simulink model "lesson140313_22"  (R2013a)
settings: Solver=ode45  StartTime=0.0  StopTime=10.0  RelTol=1e-3
settings Model: Creator=mulleda2  LastModifiedBy=mulleda2

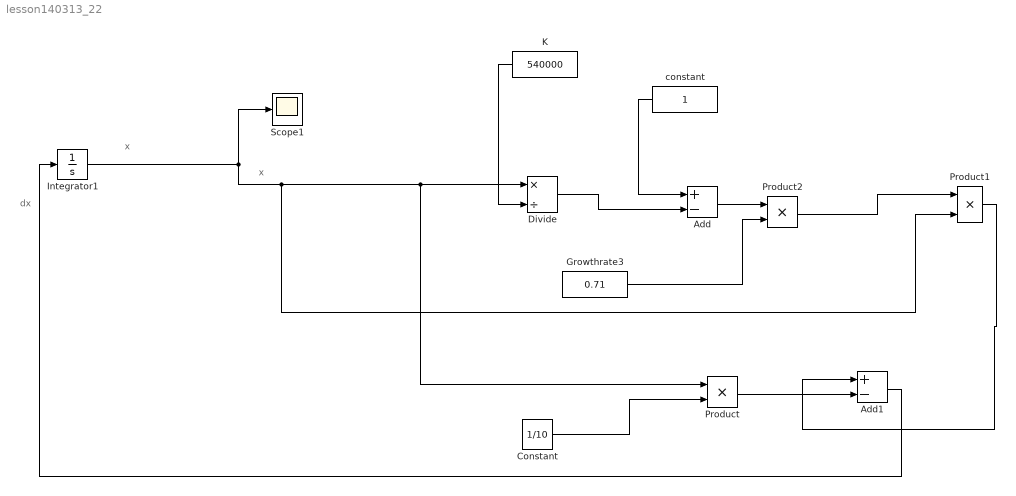
== system lesson140313_22 ==
  note: x
  note: dx
  note: x
  Add : Sum  Inputs=+-
  Add1 : Sum  Inputs=+-
  Constant : Constant  Value=1/10
  Divide : Product  Inputs=*/
  Growthrate3 : Constant  Value=0.71
  Integrator1 : Integrator  InitialCondition=540000/4
  K : Constant  Value=540000
  Product : Product
  Product1 : Product
  Product2 : Product
  Scope1 : Scope
  constant : Constant
  wires:
  Integrator1/1 -> Product1/2, Product/1, Divide/1, Scope1/1
  K/1 -> Divide/2
  constant/1 -> Add/1
  Divide/1 -> Add/2
  Add/1 -> Product2/1
  Growthrate3/1 -> Product2/2
  Product2/1 -> Product1/1
  Product1/1 -> Add1/1
  Constant/1 -> Product/2
  Product/1 -> Add1/2
  Add1/1 -> Integrator1/1
